simulink model "CenterOutReach"  (R2015b)
settings: configuration reference "CenterOutReachConfigSet" (kept outside this file)
PreLoadFcn:
  | initialize();
InitFcn:
  | initialize();
libraries: slrtlib x10, libBusSerialize x4, commfilt2 x4, simulink x2
settings Model: SimulationMode=external  Creator=djoshea  LastModifiedBy=shenoylab
settings ConfigSetRef: SourceLocation=Base Workspace

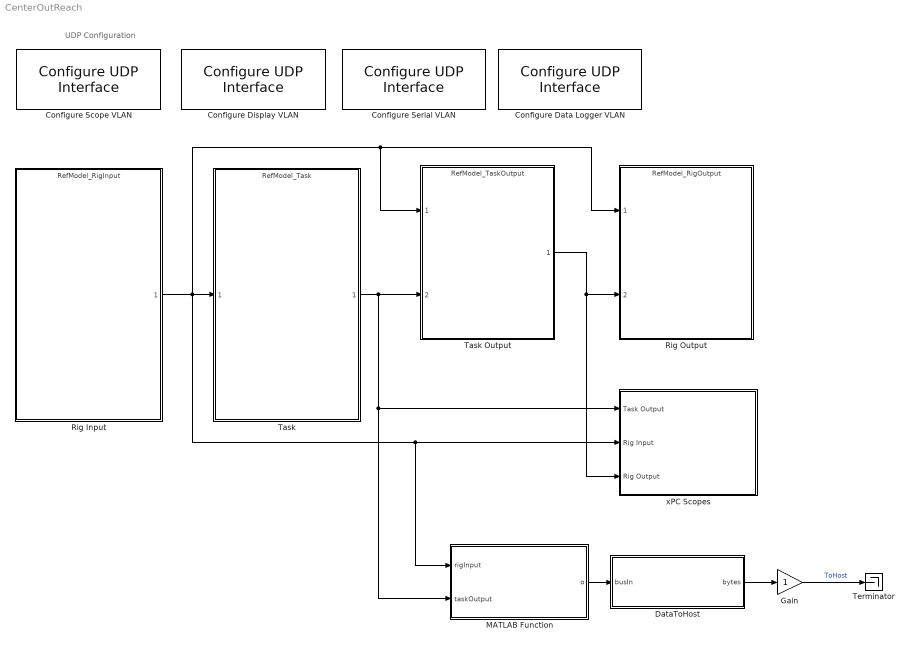
== system CenterOutReach ==
  note: UDP Configuration
  Configure Data Logger VLAN : libBusSerialize/Configure UDP Interface  PoolSizes=[100 10 10 200]  ID=RigInfo.network.dataLoggerVLAN.ethernetId  udpID=0  IpAddress=RigInfo.network.dataLoggerVLAN.sourceIP  SubnetMask=255.255.255.0  Gateway=0.0.0.0  EthDrv=Intel Gigabit  PciBus=RigInfo.network.dataLoggerVLAN.pciBus  PciSlot=RigInfo.network.dataLoggerVLAN.pciSlot
  Configure Display VLAN : libBusSerialize/Configure UDP Interface  PoolSizes=[100 10 10 200]  ID=RigInfo.network.displayVLAN.ethernetId  udpID=0  IpAddress=RigInfo.network.displayVLAN.sourceIP  SubnetMask=255.255.255.0  Gateway=0.0.0.0  EthDrv=Intel Gigabit  PciBus=RigInfo.network.displayVLAN.pciBus  PciSlot=RigInfo.network.displayVLAN.pciSlot
  Configure Scope VLAN : libBusSerialize/Configure UDP Interface  PoolSizes=[100 10 10 200]  ID=RigInfo.network.scopeVLAN.ethernetId  udpID=0  IpAddress=RigInfo.network.scopeVLAN.sourceIP  SubnetMask=255.255.255.0  Gateway=0.0.0.0  EthDrv=Intel Gigabit  PciBus=RigInfo.network.scopeVLAN.pciBus  PciSlot=RigInfo.network.scopeVLAN.pciSlot
  Configure Serial VLAN : libBusSerialize/Configure UDP Interface  PoolSizes=[100 10 10 200]  ID=RigInfo.network.serialVLAN.ethernetId  udpID=0  IpAddress=RigInfo.network.serialVLAN.sourceIP  SubnetMask=255.255.255.0  Gateway=0.0.0.0  EthDrv=Intel Gigabit  PciBus=RigInfo.network.serialVLAN.pciBus  PciSlot=RigInfo.network.serialVLAN.pciSlot
  DataToHost : MATLAB Function  AncestorBlock=libBusSerialize/Serialize  TreatAsAtomicUnit=on  mask(BusSerialize: serialize block){busType=Bus: ToHostBus}
      mask prompts: busType "Bus Type"
      mask help: Select the bus type below to serialize.
      mask init:
      | BusSerialize.maskSerializeBlockUpdate(gcb)
  Gain : Gain  ParamDataTypeStr=uint8  OutDataTypeStr=uint8
  MATLAB Function : MATLAB Function  TreatAsAtomicUnit=on
  Rig Input : ModelReference  ModelNameDialog=RefModel_RigInput.slx  SimulationMode=Normal  ModelReferenceVersion=1.362  CopyOfModelName=RefModel_RigInput.slx
  Rig Output : ModelReference  ModelNameDialog=RefModel_RigOutput.slx  SimulationMode=Normal  ModelReferenceVersion=1.189  CopyOfModelName=RefModel_RigOutput.slx
  Task : ModelReference  ModelNameDialog=RefModel_Task.slx  SimulationMode=Normal  ModelReferenceVersion=1.552  CopyOfModelName=RefModel_Task.slx
  Task Output : ModelReference  ModelNameDialog=RefModel_TaskOutput.slx  SimulationMode=Normal  ModelReferenceVersion=1.335  CopyOfModelName=RefModel_TaskOutput.slx
  Terminator : Terminator
  xPC Scopes : Subsystem
  wires:
  Task/1 -> MATLAB Function/2(taskOutput), xPC Scopes/1(Task Output), Task Output/2
  Task Output/1 -> xPC Scopes/3(Rig Output), Rig Output/2
  Rig Input/1 -> MATLAB Function/1(rigInput), xPC Scopes/2(Rig Input), Task/1, Rig Output/1, Task Output/1
  DataToHost/1(bytes) -> Gain/1
  MATLAB Function/1(o) -> DataToHost/1(busIn)
  Gain/1 -> Terminator/1  "ToHost"

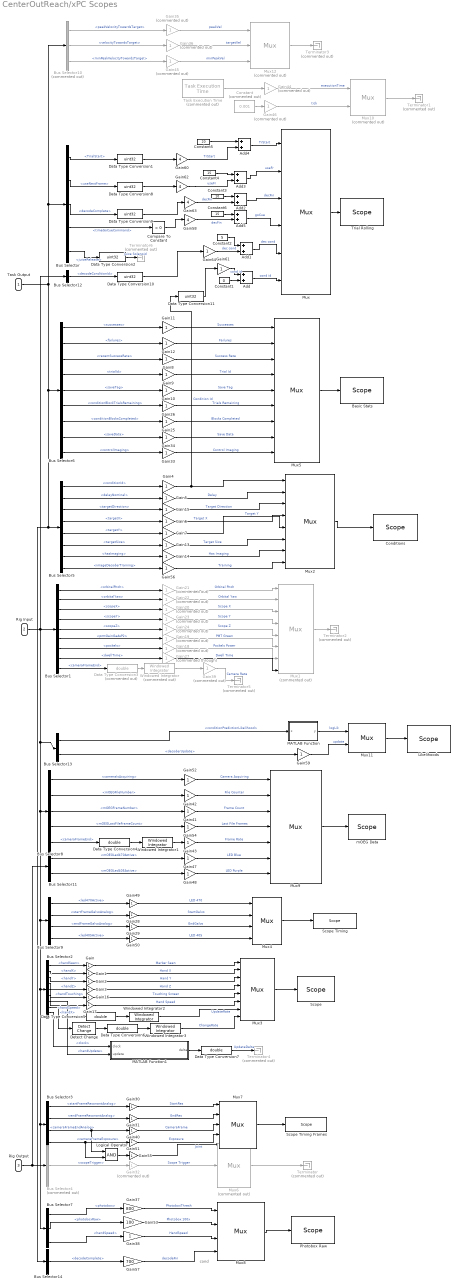
== system CenterOutReach/xPC Scopes ==
  note: cond
  note: `
  Task Output : Inport
  Rig Input : Inport  Port=2
  Rig Output : Inport  Port=3  OutDataTypeStr=Bus: RigOutputBus
  Add{,1..5} (6 alike) : Sum
  Basic Stats : slrtlib/Displays and Logging/Scope   scopeno=2  scopetype=Target  autostart=on  viewmode=Numerical  formatstr='%.0f,%.0f,%.2f,%.0f,%.0f,%.0f,%.0f,%.0f,%.0f'  grid=on  ylimits=[0,0]  nosamples=250  noprepostsamples=0  interleave=1  triggermode=FreeRun  triggersignal=1  trigsignalfromport=off  triggerlevel=0.0  triggerslope=Either  triggerscope=1  triggersample=0  filename=data.dat  mode=Lazy  writesize=512  autorestart=off  dynamicfilemode=off  maxwritefilesize=512*1024^2
  Bus Selector : BusSelector  OutputSignals=TrialStart,trialData.useNextFrame,trialData.decodeComplete,trialData.timeGoCueCommand,juiceRelease
  Bus Selector1 : BusSelector  OutputSignals=scopeState.orbitalPitch,scopeState.orbitalYaw,scopeState.scopeX,scopeState.scopeY,scopeState.scopeZ,scopeState.pmtGainGaAsP2,scopeState.pockels,scopeState.dwellTime,scopeTiming.cameraFrameEnd
  Bus Selector10 : BusSelector  Commented=on  OutputSignals=trialData.peakVelocityTowardsTarget,trialData.velocityTowardsTarget,param.minPeakVelocityTowardsTarget
  Bus Selector11 : BusSelector  OutputSignals=mOEGLed470Active,mOEGLed405Active
  Bus Selector12 : BusSelector  OutputSignals=decoderBus.decodeConditionId
  Bus Selector13 : BusSelector  OutputSignals=decoderBus.conditionPredictionLikelihood,decoderBus.decoderUpdate
  Bus Selector14 : BusSelector  OutputSignals=trialData.decodeComplete
  Bus Selector2 : BusSelector  OutputSignals=hand.handSeen,hand.handX,hand.handY,hand.handZ,hand.handTouching,hand.handSpeed,hand.handUpdate,hand.handX,clock
  Bus Selector3 : BusSelector  OutputSignals=scopeTiming.startFrameResonantAnalog,scopeTiming.endFrameResonantAnalog,scopeTiming.cameraFrameEndAnalog,scopeTiming.cameraFrameExposure
  Bus Selector4 : BusSelector  Commented=on  OutputSignals=scopeTrigger
  Bus Selector5 : BusSelector  OutputSignals=condition.conditionId,condition.delayNominal,condition.targetDirection,condition.targetX,condition.targetY,condition.targetSize,condition.hasImaging,param.imageDecoderTraining
  Bus Selector6 : BusSelector  OutputSignals=taskStatistics.successes,taskStatistics.failures,taskStatistics.recentSuccessRate,trialId,dataLoggerInfo.saveTag,taskStatistics.conditionBlockTrialsRemaining,taskStatistics.conditionBlocksCompleted,taskControl.saveData,taskControl.controlImaging
  Bus Selector7 : BusSelector  OutputSignals=analog.photobox,analog.photoboxRaw,hand.handSpeed
  Bus Selector8 : BusSelector  OutputSignals=scopeState.cameraIsAcquiring,mOEGFrameInfo.mOEGFileNumber,mOEGFrameInfo.mOEGFrameNumber,mOEGFrameInfo.mOEGLastFileFrameCount,scopeTiming.cameraFrameEnd
  Bus Selector9 : BusSelector  OutputSignals=scopeTiming.led470Active,scopeTiming.startFrameGalvoAnalog,scopeTiming.endFrameGalvoAnalog,scopeTiming.led405Active
  Compare To Constant : simulink/Logic and Bit Operations/Compare To Constant  relop=>  const=0  OutDataTypeStr=uint8
  Conditions : slrtlib/Displays and Logging/Scope   scopeno=3  scopetype=Target  autostart=on  viewmode=Numerical  formatstr='%.0f,%.0f,%.0f,%0.f,%.2f,%.2f,%.2f,%.0f'  grid=on  ylimits=[0 1000]  nosamples=2000  noprepostsamples=0  interleave=1  triggermode=FreeRun  triggersignal=1  trigsignalfromport=off  triggerlevel=0.0  triggerslope=Either  triggerscope=1  triggersample=0  filename=data.dat  mode=Lazy  writesize=512  autorestart=off  dynamicfilemode=off  maxwritefilesize=512*1024^2
  Constant : Constant  Commented=on  Value=0.001  OutDataTypeStr=double
  Constant1 : Constant  Value=0
  Constant2 : Constant  Value=5
  Constant3 : Constant  Value=10
  Constant4 : Constant  Value=15
  Constant5 : Constant  Value=20
  Constant6 : Constant  Value=15
  Data Type Conversion{1..2,8..11} (6 alike) : DataTypeConversion  OutDataTypeStr=uint32
  Data Type Conversion3 : DataTypeConversion  Commented=on  OutDataTypeStr=double
  Data Type Conversion{4..7} (4 alike) : DataTypeConversion  OutDataTypeStr=double
  Detect Change : simulink/Logic and Bit Operations/Detect Change  vinit=0  InputProcessing=Inherited  OutDataTypeStr=boolean
  Gain{,1..17,25..26,28..31,33..34,38,40..43,47..52,54..56,59,61,64} (43 alike) : Gain  OutDataTypeStr=double
  Gain{18..24,32,39} (9 alike) : Gain  Commented=on  OutDataTypeStr=double
  Gain27 : Gain  Commented=through  OutDataTypeStr=double
  Gain35 : Gain  Commented=on
  Gain36 : Gain  Commented=on
  Gain37 : Gain  Gain=800  OutDataTypeStr=double
  Gain44 : Gain  Commented=on  ParamDataTypeStr=double  OutDataTypeStr=double
  Gain45 : Gain  Commented=on
  Gain46 : Gain  Commented=on  ParamDataTypeStr=double  OutDataTypeStr=double
  Gain53 : Gain  Gain=100  OutDataTypeStr=double
  Gain57 : Gain  Gain=700  OutDataTypeStr=double
  Gain{58,60,62..63} (4 alike) : Gain  Gain=4  OutDataTypeStr=double
  Likelihoods : slrtlib/Displays and Logging/Scope   scopeno=6  scopetype=Target  autostart=on  viewmode=Graphical rolling  formatstr='%15.3f'  grid=on  ylimits=[-0.5 3]  nosamples=4000  noprepostsamples=0  interleave=1  triggermode=FreeRun  triggersignal=1  trigsignalfromport=off  triggerlevel=0.0  triggerslope=Either  triggerscope=1  triggersample=0  filename=data.dat  mode=Lazy  writesize=512  autorestart=off  dynamicfilemode=off  maxwritefilesize=512*1024^2
  Logical Operator : Logic  AllPortsSameDT=off  OutDataTypeStr=boolean
  MATLAB Function : MATLAB Function  TreatAsAtomicUnit=on
  MATLAB Function1 : MATLAB Function  TreatAsAtomicUnit=on
  Mux : Mux  Inputs=6
      settings: DisplayOption=signals
  Mux1 : Mux  Commented=on  Inputs=8
      settings: DisplayOption=signals
  Mux10 : Mux  Commented=on  Inputs=2
      settings: DisplayOption=signals
  Mux11 : Mux  Inputs=2
      settings: DisplayOption=signals
  Mux12 : Mux  Commented=on  Inputs=3
      settings: DisplayOption=signals
  Mux2 : Mux  Inputs=8
      settings: DisplayOption=signals
  Mux3 : Mux  Inputs=8
      settings: DisplayOption=signals
  Mux4 : Mux
      settings: DisplayOption=signals
  Mux5 : Mux  Inputs=9
      settings: DisplayOption=signals
  Mux6 : Mux  Commented=on  Inputs=1
      settings: DisplayOption=signals
  Mux7 : Mux  Inputs=5
      settings: DisplayOption=signals
  Mux8 : Mux
      settings: DisplayOption=signals
  Mux9 : Mux  Inputs=7
      settings: DisplayOption=signals
  Photobox Raw : slrtlib/Displays and Logging/Scope   scopeno=5  scopetype=Target  autostart=on  viewmode=Graphical rolling  formatstr='%.0f'  grid=on  ylimits=[0 1000]  nosamples=1000  noprepostsamples=0  interleave=1  triggermode=FreeRun  triggersignal=1  trigsignalfromport=off  triggerlevel=0.0  triggerslope=Either  triggerscope=1  triggersample=0  filename=data.dat  mode=Lazy  writesize=512  autorestart=off  dynamicfilemode=off  maxwritefilesize=512*1024^2
  "Scope " : slrtlib/Displays and Logging/Scope   scopeno=1  scopetype=Target  autostart=on  viewmode=Numerical  formatstr='%5.0f,%5.0f,%5.0f,%5.0f,%5.0f,%5.0f,%5.0f,%5.0f'  grid=on  ylimits=[0,0]  nosamples=250  noprepostsamples=0  interleave=1  triggermode=FreeRun  triggersignal=1  trigsignalfromport=off  triggerlevel=0.0  triggerslope=Either  triggerscope=1  triggersample=0  filename=data.dat  mode=Lazy  writesize=512  autorestart=off  dynamicfilemode=off  maxwritefilesize=512*1024^2
  Scope Timing : slrtlib/Displays and Logging/Scope   scopeno=9  scopetype=Target  autostart=on  viewmode=Graphical rolling  formatstr='%.0f'  grid=on  ylimits=[-1 6]  nosamples=1000  noprepostsamples=0  interleave=1  triggermode=FreeRun  triggersignal=1  trigsignalfromport=off  triggerlevel=0.0  triggerslope=Either  triggerscope=1  triggersample=0  filename=data.dat  mode=Lazy  writesize=512  autorestart=off  dynamicfilemode=off  maxwritefilesize=512*1024^2
  Scope Timing Frames : slrtlib/Displays and Logging/Scope   scopeno=8  scopetype=Target  autostart=on  viewmode=Graphical redraw  formatstr='%.0f'  grid=on  ylimits=[-1 6]  nosamples=250  noprepostsamples=0  interleave=1  triggermode=FreeRun  triggersignal=1  trigsignalfromport=off  triggerlevel=0.0  triggerslope=Either  triggerscope=1  triggersample=0  filename=data.dat  mode=Lazy  writesize=512  autorestart=off  dynamicfilemode=off  maxwritefilesize=512*1024^2
  "Task Execution Time " : slrtlib/Target Management/Execution Parameters/Task Execution Time   Commented=on  ts=0.001
  Terminator{,1..6} (7 alike) : Terminator  Commented=on
  Trial Rolling : slrtlib/Displays and Logging/Scope   scopeno=4  scopetype=Target  autostart=on  viewmode=Graphical rolling  formatstr='%.0f'  grid=on  ylimits=[-1 26]  nosamples=1000  noprepostsamples=0  interleave=1  triggermode=FreeRun  triggersignal=1  trigsignalfromport=off  triggerlevel=0.0  triggerslope=Either  triggerscope=1  triggersample=0  filename=data.dat  mode=Lazy  writesize=512  autorestart=off  dynamicfilemode=off  maxwritefilesize=512*1024^2
  Windowed Integrator : commfilt2/Windowed Integrator  Commented=on  integperiod=1000  roundingMode=Floor  overflowMode=off  InputProcessing=Columns as channels (frame based)
  Windowed Integrator1 : commfilt2/Windowed Integrator  integperiod=1000  roundingMode=Floor  overflowMode=off  InputProcessing=Columns as channels (frame based)
  Windowed Integrator2 : commfilt2/Windowed Integrator  integperiod=1000  roundingMode=Floor  overflowMode=off  InputProcessing=Columns as channels (frame based)
  Windowed Integrator3 : commfilt2/Windowed Integrator  integperiod=1000  roundingMode=Floor  overflowMode=off  InputProcessing=Columns as channels (frame based)
  mOEG Data : slrtlib/Displays and Logging/Scope   scopeno=7  scopetype=Target  autostart=on  viewmode=Numerical  formatstr='%.0f,%.0f,%.0f,%.0f,%.0f,%.0f,%.0f'  grid=on  ylimits=[0,0]  nosamples=250  noprepostsamples=0  interleave=1  triggermode=FreeRun  triggersignal=1  trigsignalfromport=off  triggerlevel=0.0  triggerslope=Either  triggerscope=1  triggersample=0  filename=data.dat  mode=Lazy  writesize=512  autorestart=off  dynamicfilemode=off  maxwritefilesize=512*1024^2
  wires:
  Task Output/1 -> Bus Selector10/1, Bus Selector/1, Bus Selector14/1, Bus Selector5/1, Bus Selector6/1
  Mux/1 -> Trial Rolling/1
  Bus Selector/1 -> Data Type Conversion1/1  "<TrialStart>"
  Data Type Conversion1/1 -> Gain60/1
  Bus Selector/5 -> Data Type Conversion2/1  "<juiceRelease>"
  Data Type Conversion2/1 -> Terminator6/1  "Juice Solenoid"
  Mux2/1 -> Conditions/1
  Gain4/1 -> Data Type Conversion11/1, Mux2/1  "Condition Id"
  Gain5/1 -> Mux2/2  "Delay"
  Gain6/1 -> Mux2/4  "Target X"
  Gain7/1 -> Mux2/5  "Target Y"
  Bus Selector6/1 -> Gain11/1  "<successes>"
  Mux5/1 -> Basic Stats/1
  Gain9/1 -> Mux5/4  "Trial Id"
  Gain10/1 -> Mux5/5  "Save Tag"
  Bus Selector6/3 -> Gain8/1  "<recentSuccessRate>"
  Bus Selector6/2 -> Gain12/1  "<failures>"
  Gain11/1 -> Mux5/1  "Successes"
  Gain12/1 -> Mux5/2  "Failures"
  Gain8/1 -> Mux5/3  "Success Rate"
  Gain13/1 -> Mux2/6  "Target Size"
  Gain14/1 -> Mux2/7  "Has Imaging"
  Bus Selector5/1 -> Gain4/1  "<conditionId>"
  Bus Selector5/2 -> Gain5/1  "<delayNominal>"
  Bus Selector5/4 -> Gain6/1  "<targetX>"
  Bus Selector5/5 -> Gain7/1  "<targetY>"
  Bus Selector5/6 -> Gain13/1  "<targetSize>"
  Bus Selector5/7 -> Gain14/1  "<hasImaging>"
  Gain26/1 -> Mux5/6  "Trials Remaining"
  Gain25/1 -> Mux5/7  "Blocks Completed"
  Bus Selector6/7 -> Gain25/1  "<conditionBlocksCompleted>"
  Bus Selector6/4 -> Gain9/1  "<trialId>"
  Bus Selector6/5 -> Gain10/1  "<saveTag>"
  Bus Selector6/6 -> Gain26/1  "<conditionBlockTrialsRemaining>"
  Gain34/1 -> Mux5/8  "Save Data"
  Gain33/1 -> Mux5/9  "Control Imaging"
  Bus Selector6/9 -> Gain33/1  "<controlImaging>"
  Bus Selector6/8 -> Gain34/1  "<saveData>"
  Mux12/1 -> Terminator3/1
  Bus Selector10/1 -> Gain35/1  "<peakVelocityTowardsTarget>"
  Gain35/1 -> Mux12/1  "peakVel"
  Gain36/1 -> Mux12/2  "targetVel"
  Bus Selector10/2 -> Gain36/1  "<velocityTowardsTarget>"
  "Task Execution Time "/1 -> Gain44/1
  Gain45/1 -> Mux12/3  "minPeakVel"
  Bus Selector10/3 -> Gain45/1  "<minPeakVelocityTowardsTarget>"
  Gain44/1 -> Mux10/1  "executionTime"
  Constant/1 -> Gain46/1
  Gain46/1 -> Mux10/2  "tick"
  Mux10/1 -> Terminator1/1
  Bus Selector5/3 -> Gain15/1  "<targetDirection>"
  Gain15/1 -> Mux2/3  "Target Direction"
  Bus Selector1/6 -> Gain19/1  "<pmtGainGaAsP2>"
  Bus Selector1/4 -> Gain23/1  "<scopeY>"
  Bus Selector1/7 -> Gain18/1  "<pockels>"
  Bus Selector1/5 -> Gain24/1  "<scopeZ>"
  Bus Selector1/1 -> Gain21/1  "<orbitalPitch>"
  Bus Selector1/3 -> Gain20/1  "<scopeX>"
  Bus Selector1/8 -> Gain27/1  "<dwellTime>"
  Bus Selector1/2 -> Gain22/1  "<orbitalYaw>"
  Mux3/1 -> "Scope "/1
  Gain/1 -> Mux3/1  "Marker Seen"
  Gain16/1 -> Mux3/5  "Touching Screen"
  Gain1/1 -> Mux3/2  "Hand X"
  Gain2/1 -> Mux3/3  "Hand Y"
  Gain3/1 -> Mux3/4  "Hand Z"
  Gain17/1 -> Mux3/6  "Hand Speed"
  Bus Selector2/1 -> Gain/1  "<handSeen>"
  Bus Selector2/2 -> Gain1/1  "<handX>"
  Bus Selector2/3 -> Gain2/1  "<handY>"
  Bus Selector2/4 -> Gain3/1  "<handZ>"
  Bus Selector2/5 -> Gain16/1  "<handTouching>"
  Bus Selector2/6 -> Gain17/1  "<handSpeed>"
  Gain18/1 -> Mux1/7  "Pockels Power"
  Gain21/1 -> Mux1/1  "Orbital Pitch"
  Gain22/1 -> Mux1/2  "Orbital Yaw"
  Gain20/1 -> Mux1/3  "Scope X"
  Gain23/1 -> Mux1/4  "Scope Y"
  Gain24/1 -> Mux1/5  "Scope Z"
  Gain19/1 -> Mux1/6  "PMT Green"
  Gain27/1 -> Mux1/8  "Dwell Time"
  Rig Input/1 -> Bus Selector1/1, Bus Selector7/1, Bus Selector3/1, Bus Selector2/1, Bus Selector9/1, Bus Selector8/1, Bus Selector13/1, Bus Selector12/1
  Bus Selector3/1 -> Gain30/1  "<startFrameResonantAnalog>"
  Gain30/1 -> Mux7/1  "StartRes"
  Bus Selector3/2 -> Gain31/1  "<endFrameResonantAnalog>"
  Gain31/1 -> Mux7/2  "EndRes"
  Rig Output/1 -> Bus Selector11/1, Bus Selector4/1
  Bus Selector4/1 -> Gain32/1  "<scopeTrigger>"
  Gain32/1 -> Mux6/1  "Scope Trigger"
  Mux7/1 -> Scope Timing Frames/1
  Mux6/1 -> Terminator/1
  Bus Selector7/1 -> Gain37/1  "<photobox>"
  Gain37/1 -> Mux8/1  "PhotoboxThresh"
  Mux8/1 -> Photobox Raw/1
  Bus Selector7/3 -> Gain38/1  "<handSpeed>"
  Gain38/1 -> Mux8/3  "HandSpeed"
  Data Type Conversion3/1 -> Windowed Integrator/1
  Windowed Integrator/1 -> Gain39/1
  Bus Selector1/9 -> Data Type Conversion3/1  "<cameraFrameEnd>"
  Bus Selector3/3 -> Logical Operator/1, Gain40/1  "<cameraFrameEndAnalog>"
  Gain40/1 -> Mux7/3  "CameraFrame"
  Bus Selector8/3 -> Gain41/1  "<mOEGFrameNumber>"
  Bus Selector8/4 -> Gain54/1  "<mOEGLastFileFrameCount>"
  Gain42/1 -> Mux9/2  "File Counter"
  Gain41/1 -> Mux9/3  "Frame Count"
  Windowed Integrator1/1 -> Gain43/1
  Data Type Conversion4/1 -> Windowed Integrator1/1
  Gain43/1 -> Mux9/5  "Frame Rate"
  Mux9/1 -> mOEG Data/1
  Bus Selector8/2 -> Gain42/1  "<mOEGFileNumber>"
  Bus Selector8/5 -> Data Type Conversion4/1  "<cameraFrameEnd>"
  Gain48/1 -> Mux9/7  "LED Purple"
  Gain47/1 -> Mux9/6  "LED Blue"
  Mux4/1 -> Scope Timing/1
  Bus Selector9/3 -> Gain29/1  "<endFrameGalvoAnalog>"
  Bus Selector9/2 -> Gain28/1  "<startFrameGalvoAnalog>"
  Gain29/1 -> Mux4/3  "EndGalvo"
  Gain28/1 -> Mux4/2  "StartGalvo"
  Bus Selector9/4 -> Gain50/1  "<led405Active>"
  Gain50/1 -> Mux4/4  "LED 405"
  Bus Selector9/1 -> Gain49/1  "<led470Active>"
  Gain49/1 -> Mux4/1  "LED 470"
  Gain51/1 -> Mux7/4  "Exposure"
  Bus Selector3/4 -> Logical Operator/2, Gain51/1  "<cameraFrameExposure>"
  Mux1/1 -> Terminator2/1
  Bus Selector8/1 -> Gain52/1  "<cameraIsAcquiring>"
  Gain52/1 -> Mux9/1  "Camera Acquiring"
  Bus Selector2/7 -> Data Type Conversion5/1, MATLAB Function1/2(update)  "<handUpdate>"
  Data Type Conversion5/1 -> Windowed Integrator2/1
  Windowed Integrator2/1 -> Mux3/7  "UpdateRate"
  Bus Selector2/8 -> Detect Change/1  "<handX>"
  Detect Change/1 -> Data Type Conversion6/1
  Data Type Conversion6/1 -> Windowed Integrator3/1
  Windowed Integrator3/1 -> Mux3/8  "ChangeRate"
  Bus Selector2/9 -> MATLAB Function1/1(clock)  "<clock>"
  MATLAB Function1/1(delta) -> Data Type Conversion7/1
  Data Type Conversion7/1 -> Terminator4/1  "UpdateDelta"
  Bus Selector7/2 -> Gain53/1  "<photoboxRaw>"
  Gain53/1 -> Mux8/2  "Photobox 100x"
  Gain54/1 -> Mux9/4  "Last File Frames"
  Logical Operator/1 -> Gain55/1
  Gain55/1 -> Mux7/5  "Joint"
  Bus Selector11/1 -> Gain47/1  "<mOEGLed470Active>"
  Bus Selector11/2 -> Gain48/1  "<mOEGLed405Active>"
  Bus Selector/2 -> Data Type Conversion8/1  "<useNextFrame>"
  Data Type Conversion8/1 -> Gain62/1
  Bus Selector5/8 -> Gain56/1  "<imageDecoderTraining>"
  Gain56/1 -> Mux2/8  "Training"
  Bus Selector/3 -> Data Type Conversion9/1  "<decodeComplete>"
  Data Type Conversion9/1 -> Gain63/1
  Gain39/1 -> Terminator5/1  "Camera Rate"
  Bus Selector13/1 -> MATLAB Function/1(x)  "<conditionPredictionLikelihood>"
  Mux11/1 -> Likelihoods/1
  Bus Selector13/2 -> Gain59/1  "<decoderUpdate>"
  Gain59/1 -> Mux11/2  "update"
  Bus Selector12/1 -> Data Type Conversion10/1  "<decodeConditionId>"
  Data Type Conversion10/1 -> Gain64/1
  Data Type Conversion11/1 -> Gain61/1
  Gain60/1 -> Add4/2  "TrStart"
  Gain62/1 -> Add3/2  "useFr"
  Gain63/1 -> Add2/2  "decFin"
  Gain64/1 -> Add1/2  "dec cond"
  Gain61/1 -> Add/1  "cond id"
  Constant1/1 -> Add/2
  Add/1 -> Mux/6  "cond id"
  Constant2/1 -> Add1/1
  Add1/1 -> Mux/5  "dec cond"
  Constant3/1 -> Add2/1
  Add2/1 -> Mux/3  "decFin"
  Constant4/1 -> Add3/1
  Add3/1 -> Mux/2  "useFr"
  Constant5/1 -> Add4/1
  Add4/1 -> Mux/1  "TrStart"
  MATLAB Function/1(y) -> Mux11/1  "logLik"
  Bus Selector14/1 -> Gain57/1  "<decodeComplete>"
  Gain57/1 -> Mux8/4  "decodeFin"
  Bus Selector/4 -> Compare To Constant/1  "<timeGoCueCommand>"
  Gain58/1 -> Add5/2  "decFin"
  Constant6/1 -> Add5/1
  Add5/1 -> Mux/4  "goCue"
  Compare To Constant/1 -> Gain58/1

== matlab function CenterOutReach/MATLAB Function ==
  data: rigInput input; o output Bus: ToHostBus size=1; taskOutput input; RigInfo parameter size=1
function o = buildToHost(rigInput, taskOutput, RigInfo)
%#codegen

o = initializeBus_ToHostBus();
o.rigConfig = rigInput.rigConfig;
o.clock = rigInput.clock;
o.scopeState = rigInput.scopeState;
o.juiceRelease = taskOutput.juiceRelease;
o.hand = taskOutput.handOutput;
o.eye = taskOutput.eyeOutput;
o.analog = taskOutput.analogOutput;
o.trialData = taskOutput.trialDataOutput;
o.condition = taskOutput.condition;
o.taskControl = taskOutput.taskControl;
o.param = taskOutput.param;
o.dataLoggerInfo = taskOutput.dataLoggerInfo;
o.trialId = taskOutput.trialId;
o.taskStatistics = taskOutput.taskStatistics;

bufferSize = RigInfo.outputSizes.maxEventsPerTrial;
coder.varsize('pEventBuffer', bufferSize, true);
coder.varsize('pTimestampBuffer', bufferSize, true);

persistent pEventBuffer;
persistent pTimestampBuffer;
persistent pClockTrialStart;

if isempty(pClockTrialStart)
    pClockTrialStart = rigInput.clock;
end

% initialize
if isempty(pEventBuffer) || isempty(pTimestampBuffer)
    pEventBuffer = taskOutput.taskEventQueue([], 1);
    pTimestampBuffer = zeros(0, 1, class(rigInput.clock)); %#ok<ZEROLIKE> 
    % repmat(rigInput.clock - pClockTrialStart, numel(pEventBuffer), 1);
end

if taskOutput.TrialStart
    pClockTrialStart = rigInput.clock;
    
    % clear the buffers at the start of each trial
    pEventBuffer = TaskEvent.CenterOnset;
    pTimestampBuffer = zeros(0, 1, class(rigInput.clock));  %#ok<ZEROLIKE>
end

if ~isempty(taskOutput.taskEventQueue) && numel(pEventBuffer) + numel(taskOutput.taskEventQueue) < bufferSize
%     % concatenate if no overflow
    pEventBuffer = [pEventBuffer; taskOutput.taskEventQueue];
    pTimestampBuffer = [pTimestampBuffer; repmat(rigInput.clock - pClockTrialStart, numel(taskOutput.taskEventQueue), 1)];
end

o.taskEventBuffer = pEventBuffer;
o.taskEventTimes = pTimestampBuffer;

== matlab function CenterOutReach/xPC Scopes/MATLAB Function ==
  data: x input; y output
function y = normalize(x)
% ZOH when 0, else normalize to 1.5:2.5 range
%#codegen

    persistent pY;
    if isempty(pY)
        pY = 0*x;
    end

    if ~all(isnan(x) | x == 0)
        pY = (x - nanmin(x(:))) ./ (nanmax(x(:)) - nanmin(x(:))) + 1.5;
    end
    
    y = pY;

end

== matlab function CenterOutReach/xPC Scopes/MATLAB Function1 ==
  data: clock input; delta output; update input
function delta = zohLastChangeDelta(clock, update)
%#codegen

persistent pLast;
persistent pDelta;

if isempty(pLast) || isempty(pDelta)
    pLast = zeros(1,1,'like', clock);
    pDelta = zeros(1,1,'like', clock)
end

if update
    pDelta = clock - pLast;
    pLast = clock;
end

delta = pDelta;

== matlab function CenterOutReach/DataToHost ==
  data: busIn input Bus: ToHostBus size=1; bytes output uint8 size=9193
function bytes = serialize(busIn)
%#codegen 

    bytes = serializeBus_ToHostBus(busIn);

end
